simulink library "SingleRWS"  (R2018a)
settings: Solver=ode45  StartTime=0.0  StopTime=10.0  RelTol=1e-3
undefined symbols (not defined in the file): ConfParam
libraries: simulink x1
settings Model: Creator=y.akisheva  LastModifiedBy=Cédric
settings DataIOCC: LimitDataPoints=on  SaveFormat=Array
settings OptimizationCC: BlockReduction=off  BooleanDataType=off  LifeSpan=inf
settings DebuggingCC: SaveWithParameterizedLinksMsg=none  UnderspecifiedInitializationDetection=Classic  MergeDetectMultiDrivingBlocksExec=none  SignalResolutionControl=TryResolveAllWithWarning  SFUnexpectedBacktrackingDiag=warning  SFNoUnconditionalDefaultTransitionDiag=warning  SFExecutionAtInitializationDiag=none
settings HardwareCC: ProdBitPerPointer=32  ProdBitPerSizeT=32  ProdBitPerPtrDiffT=32  ProdLargestAtomicFloat=None  ProdIntDivRoundTo=Undefined  ProdEndianess=Unspecified  ProdWordSize=32  ProdHWDeviceType=32-bit Generic  TargetUnknown=on
settings ModelReferenceCC: PropagateSignalLabelsOutOfModel=off
settings CodeAppCC: StateflowObjectComments=on
settings GRTTargetCC: TargetLangStandard=C89/C90 (ANSI)  GeneratePreprocessorConditionals=Disable all
settings ConfigComp: CovMetricSettings=dw  CovHtmlReporting=on  CovSaveCumulativeToWorkspaceVar=on  CovSaveSingleToWorkspaceVar=on  CovExternalEMLEnable=off  CovSFcnEnable=off

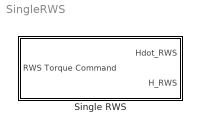
== system SingleRWS ==
  Single RWS : Subsystem

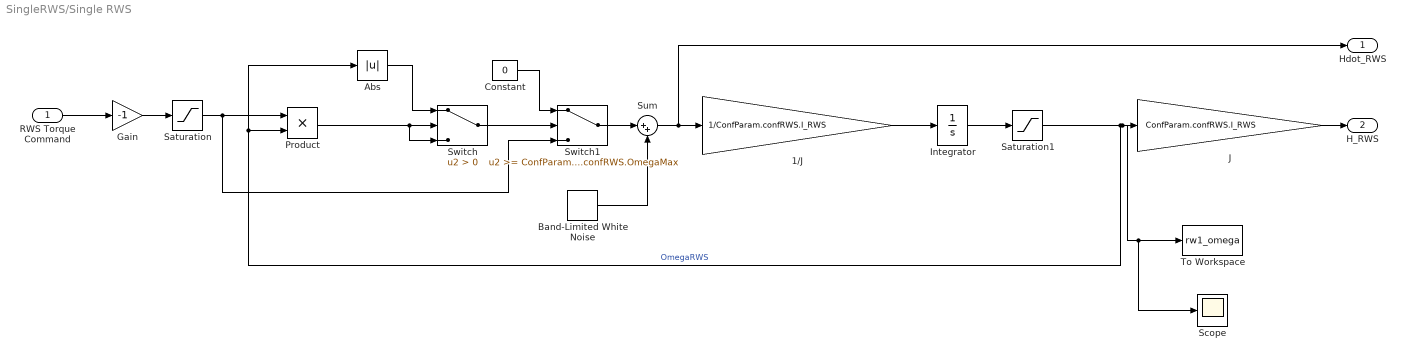
== system SingleRWS/Single RWS ==
  RWS Torque Command : Inport
  1/J : Gain  Gain=1/ConfParam.confRWS.I_RWS
  Abs : Abs
  Band-Limited White Noise : simulink/Sources/Band-Limited White Noise  Cov=ConfParam.confRWS.NoisePower  Ts=ConfParam.confOrbit.dt  seed=[23341]
  Constant : Constant  Value=0
  Gain : Gain  Gain=-1
  Integrator : Integrator  InitialCondition=ConfParam.confRWS.IntitOmegaRWS(1)
  J : Gain  Gain=ConfParam.confRWS.I_RWS
  Product : Product
  Saturation : Saturate  UpperLimit=ConfParam.confRWS.Tmax  LowerLimit=-ConfParam.confRWS.Tmax
  Saturation1 : Saturate  UpperLimit=ConfParam.confRWS.OmegaMax  LowerLimit=-ConfParam.confRWS.OmegaMax
  Scope : Scope
  Sum : Sum  Inputs=|++
  Switch : Switch  Criteria=u2 > Threshold
  Switch1 : Switch  Threshold=ConfParam.confRWS.OmegaMax
  To Workspace : ToWorkspace  VariableName=rw1_omega  SampleTime=-1
  Hdot_RWS : Outport
  H_RWS : Outport  Port=2
  wires:
  Gain/1 -> Saturation/1
  Band-Limited White Noise/1 -> Sum/2
  J/1 -> H_RWS/1
  Abs/1 -> Switch/1
  1/J/1 -> Integrator/1
  Sum/1 -> 1/J/1, Hdot_RWS/1
  Saturation1/1 -> Product/2, Abs/1, J/1, Scope/1, To Workspace/1  "OmegaRWS"
  Integrator/1 -> Saturation1/1
  Saturation/1 -> Switch1/3, Product/1
  Product/1 -> Switch/3, Switch/2
  RWS Torque Command/1 -> Gain/1
  Constant/1 -> Switch1/1
  Switch/1 -> Switch1/2
  Switch1/1 -> Sum/1
